simulink model "Hbridge"  (R2023a)
settings: Solver=VariableStepAuto  StartTime=0.0  StopTime=0.1  RelTol=1e-3
libraries: spsIGBTDiodeLib x24, spsDCVoltageSourceLib x6, simulink x4, spsThreePhaseSeriesRLCLoadLib x1, spsThreePhaseVIMeasurementLib x1, spspowerguiLib x1
settings Model: Creator=snehi  LastModifiedBy=snehi

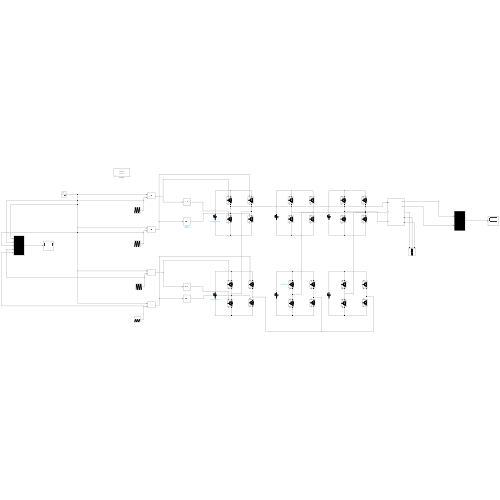
[thumbnail: Simulink's stored preview of the top-level diagram]
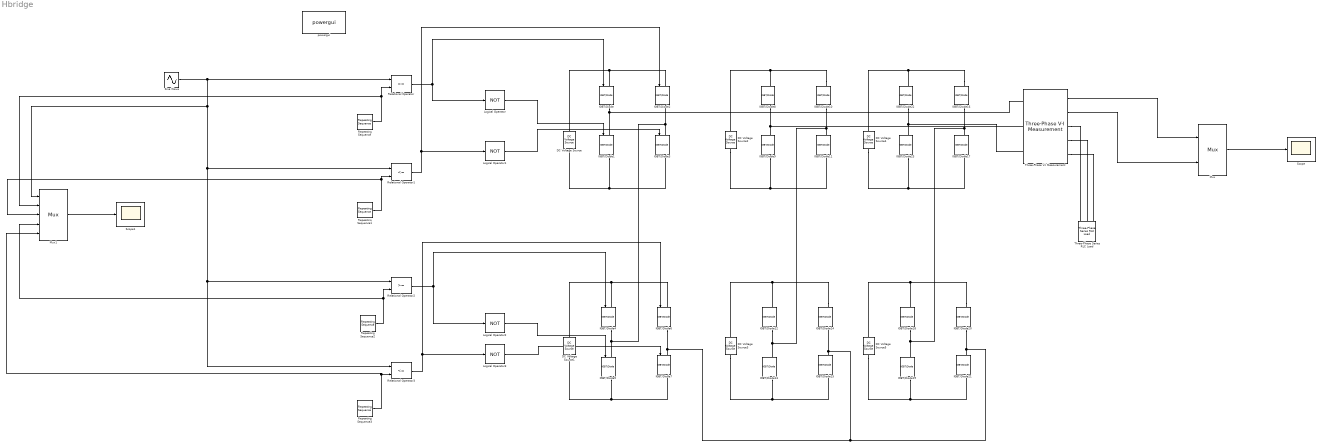
== system Hbridge ==
  DC Voltage Source{,1..5} (6 alike) : spsDCVoltageSourceLib/DC Voltage Source  Amplitude=100  Measurements=None
  IGBT/Diode{,1..23} (24 alike) : spsIGBTDiodeLib/IGBT//Diode  Ron=1e-3  Rs=1e5  Cs=inf  Measurements=on
  Logical Operator{,1..3} (4 alike) : Logic  Operator=NOT  AllPortsSameDT=off  OutDataTypeStr=boolean
  Mux : Mux  Inputs=2
  Mux1 : Mux  Inputs=5
  Relational Operator : RelationalOperator  OutDataTypeStr=boolean  RndMeth=Simplest  InputSameDT=off
  Relational Operator1 : RelationalOperator  Operator=<=  OutDataTypeStr=boolean  RndMeth=Simplest  InputSameDT=off
  Relational Operator2 : RelationalOperator  OutDataTypeStr=boolean  RndMeth=Simplest  InputSameDT=off
  Relational Operator3 : RelationalOperator  Operator=<=  OutDataTypeStr=boolean  RndMeth=Simplest  InputSameDT=off
  Repeating Sequence : simulink/Sources/Repeating Sequence  rep_seq_t=[0 0.5 1]/1000  rep_seq_y=[0.5 1 0.5]
  Repeating Sequence1 : simulink/Sources/Repeating Sequence  rep_seq_t=[0 0.5 1]/1000  rep_seq_y=[0 0.5 0]
  Repeating Sequence2 : simulink/Sources/Repeating Sequence  rep_seq_t=[0 0.5 1]/1000  rep_seq_y=[-0.5 0 -0.5]
  Repeating Sequence3 : simulink/Sources/Repeating Sequence  rep_seq_t=[0 0.5 1]/1000  rep_seq_y=[-1 -0.5 -1]
  Scope : Scope
  Scope1 : Scope
  Sine Wave : Sin  Frequency=2*pi*50  SampleTime=0
  Three-Phase Series RLC Load : spsThreePhaseSeriesRLCLoadLib/Three-Phase Series RLC Load  LConnTagsString=A|B|C  Configuration=Y (grounded)  NominalVoltage=1000  Vabc=[1e3 1e3 1e3]  Vabcp=[1e3 1e3 1e3]  NominalFrequency=60  UnbalancedPower=off  ActivePower=10e3  InductivePower=100  CapacitivePower=100  Pabc=[10e3 9e3 11e3]  QLabc=[100 90 110]  QCabc=[100 90 110]  Pabcp=[10e3 9e3 11e3]  QLabcp=[100 90 110]  QCabcp=[100 90 110]  Measurements=None  LoadType=constant Z
  Three-Phase V-I Measurement : spsThreePhaseVIMeasurementLib/Three-Phase V-I Measurement  VoltageMeasurement=phase-to-ground  SetLabelV=off  LabelV=Vabc  Vpu=off  VpuLL=off  CurrentMeasurement=yes  SetLabelI=off  LabelI=Iabc  Ipu=off  Pbase=100e6  Vbase=500e3  OutputType=Complex  PhasorSimulation=off  PSBequivalent=0
  powergui : spspowerguiLib/powergui  Priority=1  SimulationMode=Discrete  SampleTime=50e-6  frequency=60  Iterations=50  frequencyindice=0  Pbase=100e6  ErrMax=1e-4  UnitsV=kV  UnitsW=MW  buscounter=0  FunctionMessages=off  echomessages=off  EnableUseOfTLC=off  CurrentSourceSwitches=off  DisableSnubberDevices=off  DisableRonSwitches=off  DisableVfSwitches=off  DisplayEquations=off  AutomaticDiscreteSolvers=off  SolverType=Tustin/Backward Euler (TBE)  Interpol=off  ExternalGateDelay=off  methode=off  Ts=100  x0status=blocks  SPID=on  SwTol=0  HookPort=off  NonlinearTolerance=1e-4  nMaxIteration=100  ContinueOnMaxIteration=off  RestoreLinks=warning  ResistiveCurrentMeasurement=off  Frange=[0:2:500]  Ylog=off  Xlog=on  ShowGrid=off  save=off  variable=ZData  structure=0  ZoomFFT=off  StartTime=0.0  cycles=1  DisplayStyle=1  fundamental=60  FreqAxis=off  MaxFrequency=1000  frequencyindicesteady=1  RmsSteady=1  display=off
  wires:
  Repeating Sequence/1 -> Mux1/2, Relational Operator/2
  Relational Operator1/1 -> IGBT/Diode2/1, Logical Operator1/1
  Repeating Sequence1/1 -> Relational Operator1/2, Mux1/3
  Relational Operator2/1 -> IGBT/Diode4/1, Logical Operator2/1
  Repeating Sequence2/1 -> Mux1/4, Relational Operator2/2
  Relational Operator3/1 -> Logical Operator3/1, IGBT/Diode6/1
  Repeating Sequence3/1 -> Mux1/5, Relational Operator3/2
  Sine Wave/1 -> Relational Operator/1, Mux1/1, Relational Operator2/1, Relational Operator3/1, Relational Operator1/1
  Mux1/1 -> Scope1/1
  Relational Operator/1 -> IGBT/Diode/1, Logical Operator/1
  Logical Operator/1 -> IGBT/Diode1/1
  Logical Operator1/1 -> IGBT/Diode3/1
  Logical Operator2/1 -> IGBT/Diode5/1
  Logical Operator3/1 -> IGBT/Diode7/1
  Mux/1 -> Scope/1
  Three-Phase V-I Measurement/1 -> Mux/1
  Three-Phase V-I Measurement/2 -> Mux/2
  connections:
  IGBT/Diode1/LConn1 -- IGBT/Diode/RConn1 -- Three-Phase V-I Measurement/LConn1
  IGBT/Diode5/LConn1 -- IGBT/Diode4/RConn1 -- IGBT/Diode3/LConn1 -- IGBT/Diode2/RConn1
  DC Voltage Source/LConn1 -- IGBT/Diode3/RConn1 -- IGBT/Diode1/RConn1
  DC Voltage Source/RConn1 -- IGBT/Diode/LConn1 -- IGBT/Diode2/LConn1
  IGBT/Diode5/RConn1 -- IGBT/Diode7/RConn1 -- DC Voltage Source1/LConn1
  DC Voltage Source1/RConn1 -- IGBT/Diode4/LConn1 -- IGBT/Diode6/LConn1
  IGBT/Diode14/LConn1 -- DC Voltage Source3/RConn1 -- IGBT/Diode12/LConn1
  IGBT/Diode10/LConn1 -- DC Voltage Source2/RConn1 -- IGBT/Diode8/LConn1
  DC Voltage Source3/LConn1 -- IGBT/Diode13/RConn1 -- IGBT/Diode15/RConn1
  IGBT/Diode12/RConn1 -- IGBT/Diode11/LConn1 -- IGBT/Diode10/RConn1 -- IGBT/Diode13/LConn1
  IGBT/Diode9/RConn1 -- DC Voltage Source2/LConn1 -- IGBT/Diode11/RConn1
  IGBT/Diode9/LConn1 -- IGBT/Diode8/RConn1 -- Three-Phase V-I Measurement/LConn2
  Three-Phase V-I Measurement/RConn1 -- Three-Phase Series RLC Load/LConn1
  IGBT/Diode17/RConn1 -- DC Voltage Source4/LConn1 -- IGBT/Diode23/RConn1
  IGBT/Diode16/LConn1 -- DC Voltage Source4/RConn1 -- IGBT/Diode22/LConn1
  IGBT/Diode21/RConn1 -- IGBT/Diode19/RConn1 -- DC Voltage Source5/LConn1
  IGBT/Diode20/LConn1 -- DC Voltage Source5/RConn1 -- IGBT/Diode18/LConn1
  IGBT/Diode23/LConn1 -- IGBT/Diode22/RConn1 -- Three-Phase V-I Measurement/LConn3
  IGBT/Diode18/RConn1 -- IGBT/Diode17/LConn1 -- IGBT/Diode16/RConn1 -- IGBT/Diode19/LConn1
  Three-Phase V-I Measurement/RConn2 -- Three-Phase Series RLC Load/LConn2
  Three-Phase V-I Measurement/RConn3 -- Three-Phase Series RLC Load/LConn3
  IGBT/Diode21/LConn1 -- IGBT/Diode20/RConn1 -- IGBT/Diode6/RConn1 -- IGBT/Diode7/LConn1 -- IGBT/Diode14/RConn1 -- IGBT/Diode15/LConn1
